simulink model "Fig312"  (R2014b)
settings: Solver=ode3  StartTime=0.0  StopTime=10.001  FixedStep=2e-6  RelTol=1e-5
libraries: commfilt2 x1, commchan3 x1, commsink2 x1, commanapbnd3 x1, commrandsrc2 x1
settings Model: Creator=Dennis Silage  LastModifiedBy=Silage
settings DataIOCC: SignalLoggingSaveFormat=ModelDataLogs
settings OptimizationCC: ExpressionDepthLimit=2147483647  InitFltsAndDblsToZero=on
settings DebuggingCC: UnderspecifiedInitializationDetection=Classic  MergeDetectMultiDrivingBlocksExec=none  SolverPrmCheckMsg=none  FcnCallInpInsideContextMsg=UseLocalSettings  StateNameClashWarn=warning
settings GRTTargetCC: CombineOutputUpdateFcns=off  GRTInterface=on

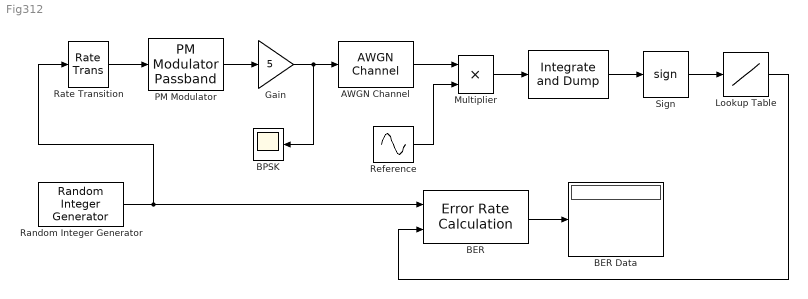
== system Fig312 ==
  " " : commfilt2/Integrate and Dump  obssamples=500  offsetsamples=0  nodump=off  roundingMode=Floor  overflowMode=off
  " Lookup Table" : Lookup_n-D  NumberOfTableDimensions=1  BreakpointsForDimension1=[-1, 0, 1]  BreakpointsForDimension3=[5, 7]  Table=[0, 0, 1]  InternalRulePriority=Speed  RndMeth=Simplest  InputSameDT=on
  AWGN Channel : commchan3/AWGN Channel  InputProcessing=Inherited (this choice will be removed - see release notes)  seed=randseed  noiseMode="Signal to noise ratio  (Eb/No)"  EbNodB=50  EsNodB=10  SNRdB=12  bitsPerSym=1  Ps=12.5  Tsym=1e-3  variance=0
  BER : commsink2/Error Rate Calculation  N=2  st_delay=0  cp_mode=Entire frame  subframe=[]  PMode=Port  WsName=ErrorVec  RsMode2=off  stop=off  numErr=100  maxBits=1e6
  BER Data : Display
  BPSK : Scope
      settings: YMin=-6  YMax=6
  Gain : Gain  Gain=5
  Multiplier : Product  RndMeth=Zero
  PM Modulator : commanapbnd3/PM Modulator Passband  Fc=20000  Ph=pi  Kc=pi
  Random Integer Generator : commrandsrc2/Random Integer Generator  mul=2  seed=randseed  Ts=1e-3  frameBased=off  sampPerFrame=50  orient=on  outDataType=double
  Rate Transition : RateTransition  OutPortSampleTime=2e-6
  Reference : Sin  Amplitude=5  Frequency=40000*pi  Phase=pi/2  Samples=200  SampleTime=2e-6
  Sign : Signum
  wires:
  Sign/1 -> " Lookup Table"/1
  BER/1 -> BER Data/1
  Multiplier/1 -> " "/1
  " "/1 -> Sign/1
  AWGN Channel/1 -> Multiplier/1
  Random Integer Generator/1 -> Rate Transition/1, BER/1
  Reference/1 -> Multiplier/2
  Gain/1 -> AWGN Channel/1, BPSK/1
  Rate Transition/1 -> PM Modulator/1
  PM Modulator/1 -> Gain/1
  " Lookup Table"/1 -> BER/2
